simulink model "jiang"  (Simulink 7.9)
settings: Solver=ode3  StartTime=0.0  StopTime=1000  FixedStep=0.05  RelTol=1e-3
libraries: simulink x3
settings Model: Creator=Staciej  LastModifiedBy=Staciej  CovModelRefEnable=off
settings DataIOCC: LimitDataPoints=off  SaveFormat=StructureWithTime  SignalLoggingSaveFormat=Dataset
settings OptimizationCC: ExpressionDepthLimit=128
settings DebuggingCC: UnderspecifiedInitializationDetection=Simplified  MergeDetectMultiDrivingBlocksExec=error  SolverPrmCheckMsg=none  FrameProcessingCompatibilityMsg=error  StateNameClashWarn=none
settings HardwareCC: ProdBitPerPointer=64  ProdLargestAtomicFloat=Float  ProdIntDivRoundTo=Zero  ProdEndianess=LittleEndian  ProdHWDeviceType=Specified
settings ModelReferenceCC: PropagateSignalLabelsOutOfModel=on
settings CodeAppCC: CustomSymbolStrType=$N$R$M_T
settings GRTTargetCC: CodeReplacementLibrary=C89/C90 (ANSI)

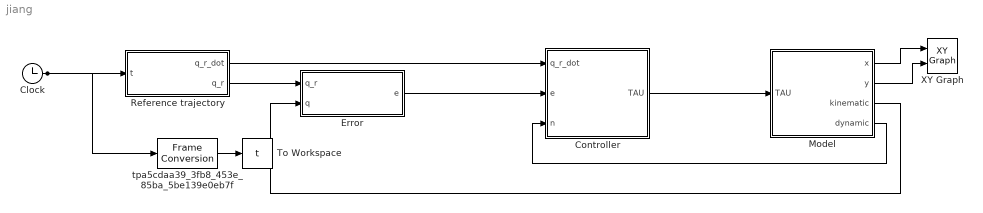
== system jiang ==
  Clock : Clock
  Controller : Subsystem
  Error : Subsystem
  Model : Subsystem
  Reference trajectory : Subsystem
  To Workspace : ToWorkspace  VariableName=t  SampleTime=-1
  XY Graph : simulink/Sinks/XY Graph  xmin=-100  xmax=1000  ymin=-200  ymax=200  st=-1
  tpa5cdaa39_3fb8_453e_85ba_5be139e0eb7f : FrameConversion  InheritSamplingMode=off  OutFrame=Sample-based
  wires:
  Clock/1 -> Reference trajectory/1(t), tpa5cdaa39_3fb8_453e_85ba_5be139e0eb7f/1
  Controller/1(TAU) -> Model/1(TAU)
  Model/1(x) -> XY Graph/1
  Model/2(y) -> XY Graph/2
  Reference trajectory/2(q_r) -> Error/1(q_r)
  Error/1(e) -> Controller/2(e)
  Model/4(dynamic) -> Controller/3(n)
  Model/3(kinematic) -> Error/2(q)
  Reference trajectory/1(q_r_dot) -> Controller/1(q_r_dot)
  tpa5cdaa39_3fb8_453e_85ba_5be139e0eb7f/1 -> To Workspace/1

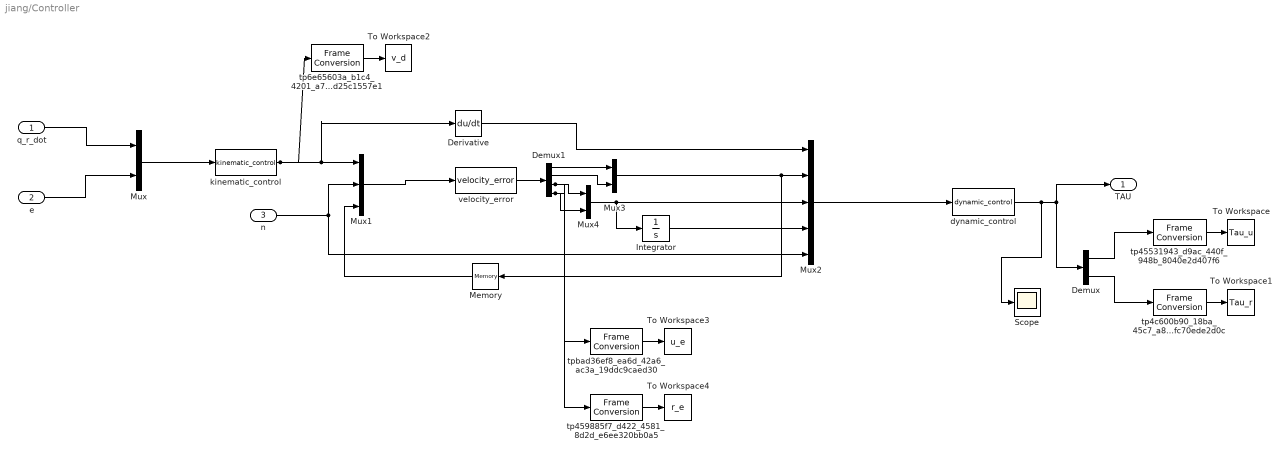
== system jiang/Controller ==
  q_r_dot : Inport
  e : Inport  Port=2
  n : Inport  Port=3
  Demux : Demux  Outputs=2
  Demux1 : Demux
  Derivative : Derivative
  Integrator : Integrator
  Memory : Memory  X0=[0;0]
  Mux : Mux  Inputs=2
  Mux1 : Mux  Inputs=3
  Mux2 : Mux  Inputs=5
  Mux3 : Mux  Inputs=2
  Mux4 : Mux  Inputs=2
  Scope : Scope
      settings: TimeRange=auto  MaxDataPoints=5000  SaveToWorkspace=off  SaveName=ScopeData  YMin=-249.84575  YMax=752.27677  SampleTime=-1
  To Workspace : ToWorkspace  VariableName=Tau_u  SampleTime=-1
  To Workspace1 : ToWorkspace  VariableName=Tau_r  SampleTime=-1
  To Workspace2 : ToWorkspace  VariableName=v_d  SampleTime=-1
  To Workspace3 : ToWorkspace  VariableName=u_e  SampleTime=-1
  To Workspace4 : ToWorkspace  VariableName=r_e  SampleTime=-1
  dynamic_control : MATLABFcn  MATLABFcn=dynamic_control  OutputDimensions=2
  kinematic_control : MATLABFcn  MATLABFcn=kinematic_control  OutputDimensions=2
  tp45531943_d9ac_440f_948b_8040e2d407f6 : FrameConversion  InheritSamplingMode=off  OutFrame=Sample-based
  tp459885f7_d422_4581_8d2d_e6ee320bb0a5 : FrameConversion  InheritSamplingMode=off  OutFrame=Sample-based
  tp4c600b90_18ba_45c7_a8fa_2fc70ede2d0c : FrameConversion  InheritSamplingMode=off  OutFrame=Sample-based
  tp6e65603a_b1c4_4201_a758_92d25c1557e1 : FrameConversion  InheritSamplingMode=off  OutFrame=Sample-based
  tpbad36ef8_ea6d_42a6_ac3a_19ddc9caed30 : FrameConversion  InheritSamplingMode=off  OutFrame=Sample-based
  velocity_error : MATLABFcn  MATLABFcn=velocity_error  OutputDimensions=4
  TAU : Outport
  wires:
  dynamic_control/1 -> Scope/1, Demux/1, TAU/1
  q_r_dot/1 -> Mux/1
  e/1 -> Mux/2
  Mux/1 -> kinematic_control/1
  kinematic_control/1 -> Derivative/1, Mux1/1, tp6e65603a_b1c4_4201_a758_92d25c1557e1/1
  Mux1/1 -> velocity_error/1
  n/1 -> Mux1/2, Mux2/5
  velocity_error/1 -> Demux1/1
  Demux1/1 -> Mux3/1
  Demux1/2 -> Mux3/2
  Mux3/1 -> Memory/1, Mux2/2
  Demux1/3 -> Mux4/1, tpbad36ef8_ea6d_42a6_ac3a_19ddc9caed30/1
  Demux1/4 -> Mux4/2, tp459885f7_d422_4581_8d2d_e6ee320bb0a5/1
  Mux4/1 -> Mux2/3, Integrator/1
  Integrator/1 -> Mux2/4
  Derivative/1 -> Mux2/1
  Mux2/1 -> dynamic_control/1
  Memory/1 -> Mux1/3
  Demux/1 -> tp45531943_d9ac_440f_948b_8040e2d407f6/1
  tp45531943_d9ac_440f_948b_8040e2d407f6/1 -> To Workspace/1
  Demux/2 -> tp4c600b90_18ba_45c7_a8fa_2fc70ede2d0c/1
  tp4c600b90_18ba_45c7_a8fa_2fc70ede2d0c/1 -> To Workspace1/1
  tp6e65603a_b1c4_4201_a758_92d25c1557e1/1 -> To Workspace2/1
  tpbad36ef8_ea6d_42a6_ac3a_19ddc9caed30/1 -> To Workspace3/1
  tp459885f7_d422_4581_8d2d_e6ee320bb0a5/1 -> To Workspace4/1

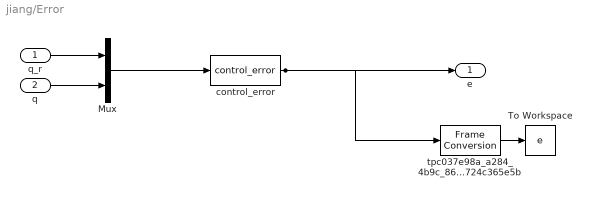
== system jiang/Error ==
  q_r : Inport
  q : Inport  Port=2
  Mux : Mux  Inputs=2
  To Workspace : ToWorkspace  VariableName=e  SampleTime=-1
  control_error : MATLABFcn  MATLABFcn=control_error  OutputDimensions=3
  tpc037e98a_a284_4b9c_8697_c0724c365e5b : FrameConversion  InheritSamplingMode=off  OutFrame=Sample-based
  e : Outport
  wires:
  q_r/1 -> Mux/1
  Mux/1 -> control_error/1
  q/1 -> Mux/2
  control_error/1 -> e/1, tpc037e98a_a284_4b9c_8697_c0724c365e5b/1
  tpc037e98a_a284_4b9c_8697_c0724c365e5b/1 -> To Workspace/1

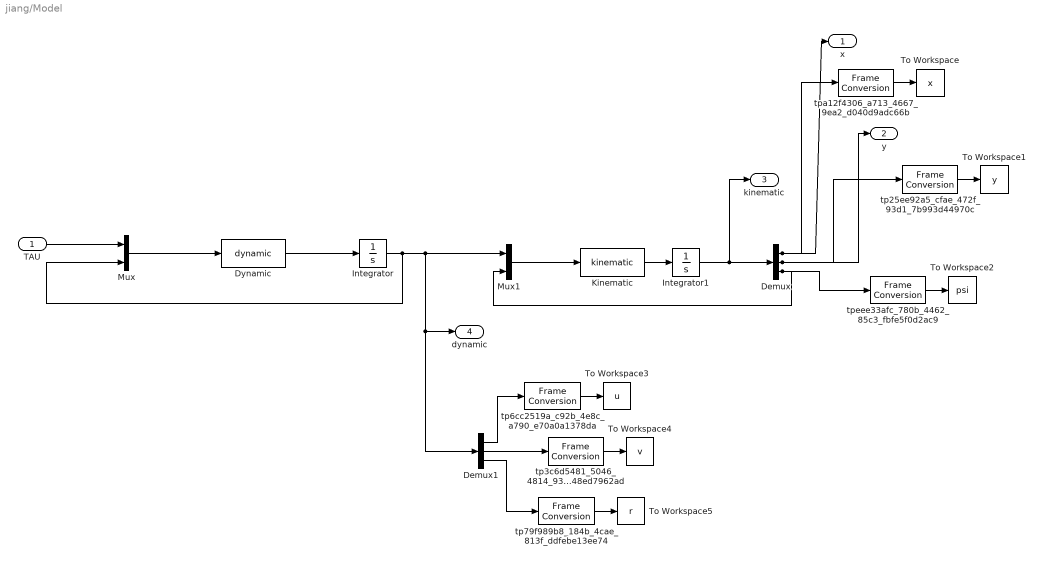
== system jiang/Model ==
  TAU : Inport
  Demux : Demux  Outputs=3
  Demux1 : Demux  Outputs=3
  Dynamic : MATLABFcn  MATLABFcn=dynamic  OutputDimensions=3
  Integrator : Integrator  InitialCondition=[0 0 0]
  Integrator1 : Integrator  InitialCondition=[5 10 0.5]
  Kinematic : MATLABFcn  MATLABFcn=kinematic  OutputDimensions=3
  Mux : Mux  Inputs=2
  Mux1 : Mux  Inputs=2
  To Workspace : ToWorkspace  VariableName=x  SampleTime=-1
  To Workspace1 : ToWorkspace  VariableName=y  SampleTime=-1
  To Workspace2 : ToWorkspace  VariableName=psi  SampleTime=-1
  To Workspace3 : ToWorkspace  VariableName=u  SampleTime=-1
  To Workspace4 : ToWorkspace  VariableName=v  SampleTime=-1
  To Workspace5 : ToWorkspace  VariableName=r  SampleTime=-1
  tp25ee92a5_cfae_472f_93d1_7b993d44970c : FrameConversion  InheritSamplingMode=off  OutFrame=Sample-based
  tp3c6d5481_5046_4814_9362_4848ed7962ad : FrameConversion  InheritSamplingMode=off  OutFrame=Sample-based
  tp6cc2519a_c92b_4e8c_a790_e70a0a1378da : FrameConversion  InheritSamplingMode=off  OutFrame=Sample-based
  tp79f989b8_184b_4cae_813f_ddfebe13ee74 : FrameConversion  InheritSamplingMode=off  OutFrame=Sample-based
  tpa12f4306_a713_4667_9ea2_d040d9adc66b : FrameConversion  InheritSamplingMode=off  OutFrame=Sample-based
  tpeee33afc_780b_4462_85c3_fbfe5f0d2ac9 : FrameConversion  InheritSamplingMode=off  OutFrame=Sample-based
  x : Outport
  y : Outport  Port=2
  kinematic : Outport  Port=3
  dynamic : Outport  Port=4
  wires:
  TAU/1 -> Mux/1
  Mux/1 -> Dynamic/1
  Dynamic/1 -> Integrator/1
  Integrator/1 -> Mux/2, Demux1/1, dynamic/1, Mux1/1
  Mux1/1 -> Kinematic/1
  Kinematic/1 -> Integrator1/1
  Demux/3 -> Mux1/2, tpeee33afc_780b_4462_85c3_fbfe5f0d2ac9/1
  Demux/1 -> x/1, tpa12f4306_a713_4667_9ea2_d040d9adc66b/1
  Demux/2 -> y/1, tp25ee92a5_cfae_472f_93d1_7b993d44970c/1
  Integrator1/1 -> kinematic/1, Demux/1
  tpa12f4306_a713_4667_9ea2_d040d9adc66b/1 -> To Workspace/1
  tp25ee92a5_cfae_472f_93d1_7b993d44970c/1 -> To Workspace1/1
  tpeee33afc_780b_4462_85c3_fbfe5f0d2ac9/1 -> To Workspace2/1
  Demux1/1 -> tp6cc2519a_c92b_4e8c_a790_e70a0a1378da/1
  tp6cc2519a_c92b_4e8c_a790_e70a0a1378da/1 -> To Workspace3/1
  Demux1/2 -> tp3c6d5481_5046_4814_9362_4848ed7962ad/1
  tp3c6d5481_5046_4814_9362_4848ed7962ad/1 -> To Workspace4/1
  Demux1/3 -> tp79f989b8_184b_4cae_813f_ddfebe13ee74/1
  tp79f989b8_184b_4cae_813f_ddfebe13ee74/1 -> To Workspace5/1

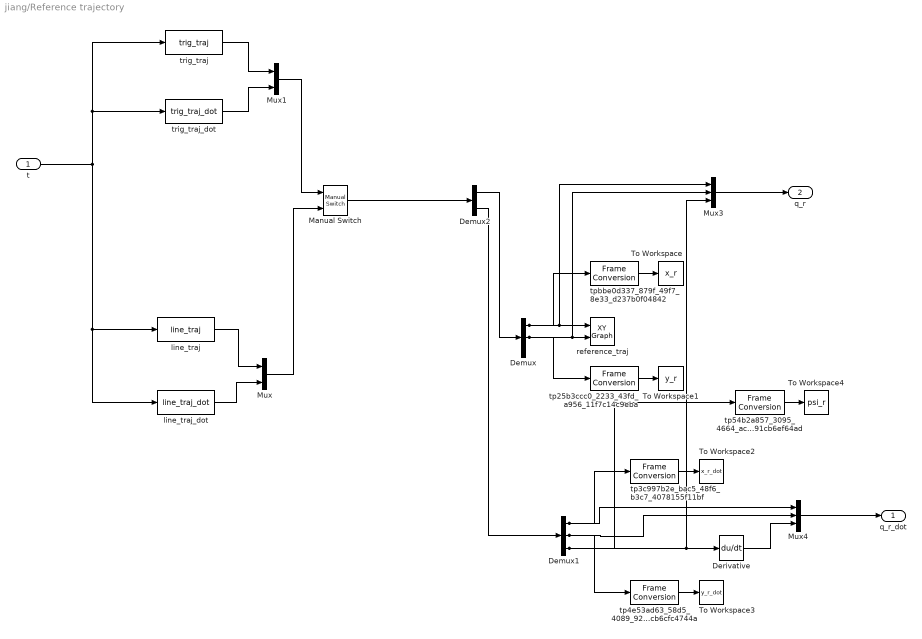
== system jiang/Reference trajectory ==
  t : Inport
  Demux : Demux  Outputs=3
  Demux1 : Demux  Outputs=3
  Demux2 : Demux  Outputs=2
  Derivative : Derivative
  Manual Switch : simulink/Signal Routing/Manual Switch  sw=1  action=0  varsize=off
  Mux : Mux  Inputs=2
  Mux1 : Mux  Inputs=2
  Mux3 : Mux  Inputs=3
  Mux4 : Mux  Inputs=3
  To Workspace : ToWorkspace  VariableName=x_r  SampleTime=-1
  To Workspace1 : ToWorkspace  VariableName=y_r  SampleTime=-1
  To Workspace2 : ToWorkspace  VariableName=x_r_dot  SampleTime=-1
  To Workspace3 : ToWorkspace  VariableName=y_r_dot  SampleTime=-1
  To Workspace4 : ToWorkspace  VariableName=psi_r  SampleTime=-1
  line_traj : MATLABFcn  MATLABFcn=line_traj  OutputDimensions=3
  line_traj_dot : MATLABFcn  MATLABFcn=line_traj_dot  OutputDimensions=3
  reference_traj : simulink/Sinks/XY Graph  xmin=-100  xmax=1000  ymin=-200  ymax=200  st=-1
  tp25b3ccc0_2233_43fd_a956_11f7c14c9eba : FrameConversion  InheritSamplingMode=off  OutFrame=Sample-based
  tp3c997b2e_bac5_48f6_b3c7_4078155f11bf : FrameConversion  InheritSamplingMode=off  OutFrame=Sample-based
  tp4e53ad63_58d5_4089_92ec_1cb6cfc4744a : FrameConversion  InheritSamplingMode=off  OutFrame=Sample-based
  tp54b2a857_3095_4664_acd4_a91cb6ef64ad : FrameConversion  InheritSamplingMode=off  OutFrame=Sample-based
  tpbbe0d337_879f_49f7_8e33_d237b0f04842 : FrameConversion  InheritSamplingMode=off  OutFrame=Sample-based
  trig_traj : MATLABFcn  MATLABFcn=trig_traj  OutputDimensions=3
  trig_traj_dot : MATLABFcn  MATLABFcn=trig_traj_dot  OutputDimensions=3
  q_r_dot : Outport
  q_r : Outport  Port=2
  wires:
  t/1 -> trig_traj_dot/1, trig_traj/1, line_traj/1, line_traj_dot/1
  Demux/1 -> reference_traj/1, Mux3/1, tpbbe0d337_879f_49f7_8e33_d237b0f04842/1
  Demux/2 -> Mux3/2, reference_traj/2, tp25b3ccc0_2233_43fd_a956_11f7c14c9eba/1
  Demux1/1 -> Mux4/1, tp3c997b2e_bac5_48f6_b3c7_4078155f11bf/1
  Demux1/2 -> Mux4/2, tp4e53ad63_58d5_4089_92ec_1cb6cfc4744a/1
  Demux2/2 -> Demux1/1
  line_traj_dot/1 -> Mux/2
  line_traj/1 -> Mux/1
  Mux/1 -> Manual Switch/2
  Demux2/1 -> Demux/1
  trig_traj_dot/1 -> Mux1/2
  trig_traj/1 -> Mux1/1
  Mux1/1 -> Manual Switch/1
  Manual Switch/1 -> Demux2/1
  Demux1/3 -> Derivative/1, Mux3/3, tp54b2a857_3095_4664_acd4_a91cb6ef64ad/1
  Derivative/1 -> Mux4/3
  Mux4/1 -> q_r_dot/1
  Mux3/1 -> q_r/1
  tpbbe0d337_879f_49f7_8e33_d237b0f04842/1 -> To Workspace/1
  tp25b3ccc0_2233_43fd_a956_11f7c14c9eba/1 -> To Workspace1/1
  tp3c997b2e_bac5_48f6_b3c7_4078155f11bf/1 -> To Workspace2/1
  tp4e53ad63_58d5_4089_92ec_1cb6cfc4744a/1 -> To Workspace3/1
  tp54b2a857_3095_4664_acd4_a91cb6ef64ad/1 -> To Workspace4/1
